simulink model "c1_chirp_filter"  (R2020b)
settings: Solver=FixedStepDiscrete  StartTime=0.0  StopTime=stopTime  FixedStep=2.0833333333333333e-05  RelTol=1e-3
values from neighbouring files (symbols this model uses):
  norm_gainc1 = (sqrt(C1gain_norm))/((sqrt(CF^2+rzero^2))^order_of_zero)    [c1_chirp_parameter.m]
undefined symbols (not defined in the file or in its folder): cihc
settings Model: Creator=Ross  LastModifiedBy=conno
settings DataIOCC: SaveOutput=off  SaveTime=off  ReturnWorkspaceOutputs=off
settings OptimizationCC: BlockReduction=off  ConditionallyExecuteInputs=off  DefaultParameterBehavior=Inlined
settings DebuggingCC: ReadBeforeWriteMsg=DisableAll  WriteAfterWriteMsg=DisableAll  WriteAfterReadMsg=DisableAll  AlgebraicLoopMsg=error  MultiTaskDSMMsg=none  SingleTaskRateTransMsg=error  PregeneratedLibrarySubsystemCodeDiagnostic=none  ArithmeticOperatorsInVariantConditions=warning
settings HardwareCC: ProdBitPerPointer=32  ProdBitPerSizeT=32  ProdBitPerPtrDiffT=32  ProdLargestAtomicFloat=None  ProdIntDivRoundTo=Undefined  ProdEndianess=Unspecified  ProdWordSize=32  ProdHWDeviceType=ASIC/FPGA->ASIC/FPGA  TargetBitPerPointer=64  TargetBitPerSizeT=64  TargetBitPerPtrDiffT=64  TargetLongLongMode=on  TargetIntDivRoundTo=Zero  TargetEndianess=LittleEndian  TargetWordSize=64  TargetHWDeviceType=Custom Processor->MATLAB Host Computer  ProdEqTarget=off
settings ModelReferenceCC: UpdateModelReferenceTargets=IfOutOfDate  ModelReferenceNumInstancesAllowed=Single
settings SFSimCC: SFSimEcho=off  SimUseLocalCustomCode=off  CustomCodeUndefinedFunction=UseInterfaceOnly
settings RTWCC: RTWUseLocalCustomCode=off

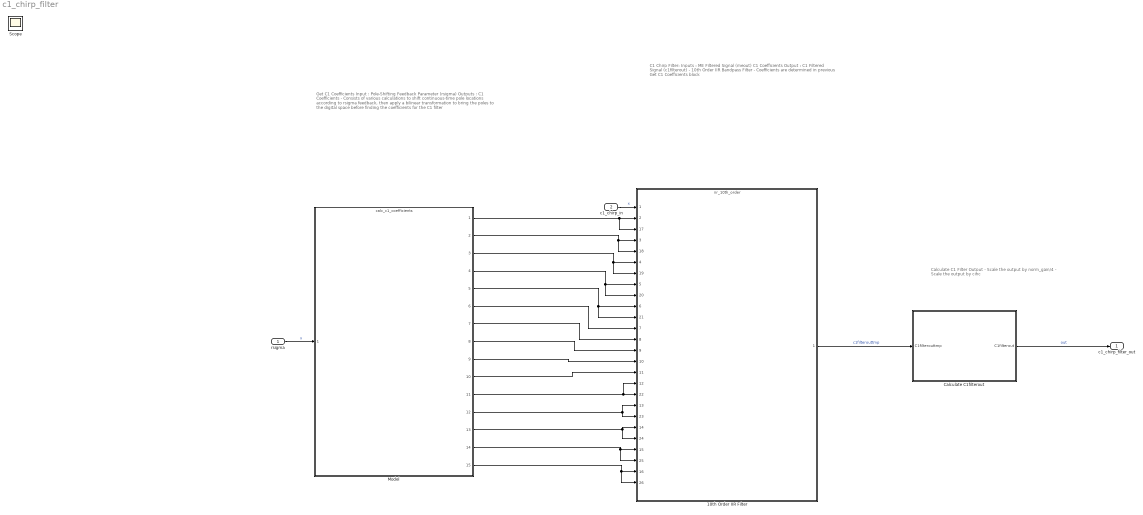
== system c1_chirp_filter ==
  note: Calculate C1 Filter Output
      | - Scale the output by norm_gain/4
      | - Scale the output by cihc
  note: Get C1 Coefficients
      |
      | Input : Pole-Shifting Feedback Parameter (rsigma)
      |
      | Outputs : C1 Coefficients
      |
      | - Consists of various calculations to shift continuous-time pole locations according to rsigma feedback, then apply a bilinear transformation to bring the poles to the digital space before finding the coefficients for the C1 filter
  note: C1 Chirp Filter:
      |
      | Inputs : ME Filtered Signal (meout)
      | C1 Coefficients
      |
      | Output : C1 Filtered Signal (c1filterout)
      |
      | - 10th Order IIR Bandpass Filter
      |
      | - Coefficients are determined in previous Get C1 Coefficients block
  rsigma : Inport  OutDataTypeStr=single  PortDimensions=1  SampleTime=[2.0833333333333333e-05,0]
  c1_chirp_in : Inport  Port=2  OutDataTypeStr=single  PortDimensions=1  SampleTime=[2.0833333333333333e-05,0]
  10th Order IIR Filter : ModelReference  ModelNameDialog=iir_10th_order  SimulationMode=Normal  ModelReferenceVersion=1.115
      settings: PortSchema="{\"entries\":[{\"content\":{\"sides\":[{\"content\":{\"connectorIds\":[\"In1\",\"In2\",\"In17\",\"In3\",\"In18\",\"In4\",\"In19\",\"In5\",\"In20\",\"In6\",\"In21\",\"In7\",\"In8\",\"In9\",\"In10\",\"In11\",\"In12\",\"In22\",\"In13\",\"In23\",\"In14\",\"In24\",\"In15\",\"In25\",\"In16\",\"In26\"]},\"type\":\"ConnectorPlacement.EquallySpacedRectSide\",\"uuid\":\"3f4bdb5d-b42d-4634-9b19-7b113449438c\"},{\"content\":{\"connectorIds\":[\"Out1\"],\"side\":\"RIGHT\"},\"type\":\"ConnectorPlacement.EquallySpacedRectSide\",\"uuid\":\"b7f66fd0-cf87-477c-ae9b-33c7ff0d8e95\"},{\"content\":{\"connectorIds\":[],\"side\":\"TOP\"},\"type\":\"ConnectorPlacement.EquallySpacedRectSide\",\"uuid\":\"4bdc3f67-4ae3-4540-9fbd-a4b9cbe08a98\"},{\"content\":{\"connectorIds\":[],\"side\":\"HIDDEN\"},\"type\":\"ConnectorPlacement.EquallySpacedRectSide\",\"uuid\":\"e88c75d7-98e2-4c6b-baaa-8b1b576ddbd9\"}]},\"type\":\"ConnectorPlacement.EquallySpacedConnector\",\"uuid\":\"8fb96455-c89c-4600-b826-8fa2bd22e05b\"}],\"packageUris\":[\"http://schema.mathworks.com/mf0/Connector/R2020b\"],\"version\":\"1.0\"}"
  Calculate C1filterout : Subsystem
  Model : ModelReference  ModelNameDialog=calc_c1_coefficients.slx  SimulationMode=Normal  ModelReferenceVersion=1.151
  c1_chirp_filter_out : Outport  OutDataTypeStr=single  PortDimensions=1  SampleTime=[2.0833333333333333e-05,0]  VectorParamsAs1DForOutWhenUnconnected=off
  Scope : Scope
  wires:
  10th Order IIR Filter/1 -> Calculate C1filterout/1(C1filterouttmp)  "c1filterouttmp"
  rsigma/1 -> Model/1  "x"
  c1_chirp_in/1 -> 10th Order IIR Filter/1  "x"
  Calculate C1filterout/1(C1filterout) -> c1_chirp_filter_out/1  "out"
  Model/1 -> 10th Order IIR Filter/17, 10th Order IIR Filter/2
  Model/2 -> 10th Order IIR Filter/18, 10th Order IIR Filter/3
  Model/3 -> 10th Order IIR Filter/19, 10th Order IIR Filter/4
  Model/4 -> 10th Order IIR Filter/20, 10th Order IIR Filter/5
  Model/5 -> 10th Order IIR Filter/21, 10th Order IIR Filter/6
  Model/6 -> 10th Order IIR Filter/7
  Model/7 -> 10th Order IIR Filter/8
  Model/8 -> 10th Order IIR Filter/9
  Model/9 -> 10th Order IIR Filter/10
  Model/10 -> 10th Order IIR Filter/11
  Model/11 -> 10th Order IIR Filter/12, 10th Order IIR Filter/22
  Model/12 -> 10th Order IIR Filter/23, 10th Order IIR Filter/13
  Model/13 -> 10th Order IIR Filter/24, 10th Order IIR Filter/14
  Model/14 -> 10th Order IIR Filter/15, 10th Order IIR Filter/25
  Model/15 -> 10th Order IIR Filter/16, 10th Order IIR Filter/26

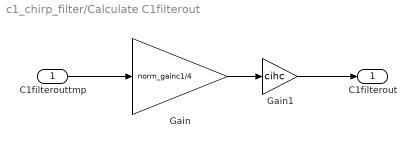
== system c1_chirp_filter/Calculate C1filterout ==
  C1filterouttmp : Inport
  Gain : Gain  Gain=norm_gainc1/4
  Gain1 : Gain  Gain=cihc
  C1filterout : Outport  VectorParamsAs1DForOutWhenUnconnected=off
  wires:
  Gain1/1 -> C1filterout/1
  Gain/1 -> Gain1/1
  C1filterouttmp/1 -> Gain/1
